simulink model "robot"  (R2017b)
settings: Solver=VariableStepAuto  StartTime=0.0  StopTime=10.0  RelTol=1e-3
libraries: vexarmcortexlib x16
settings Model: Creator=Chase B  LastModifiedBy=Chase B

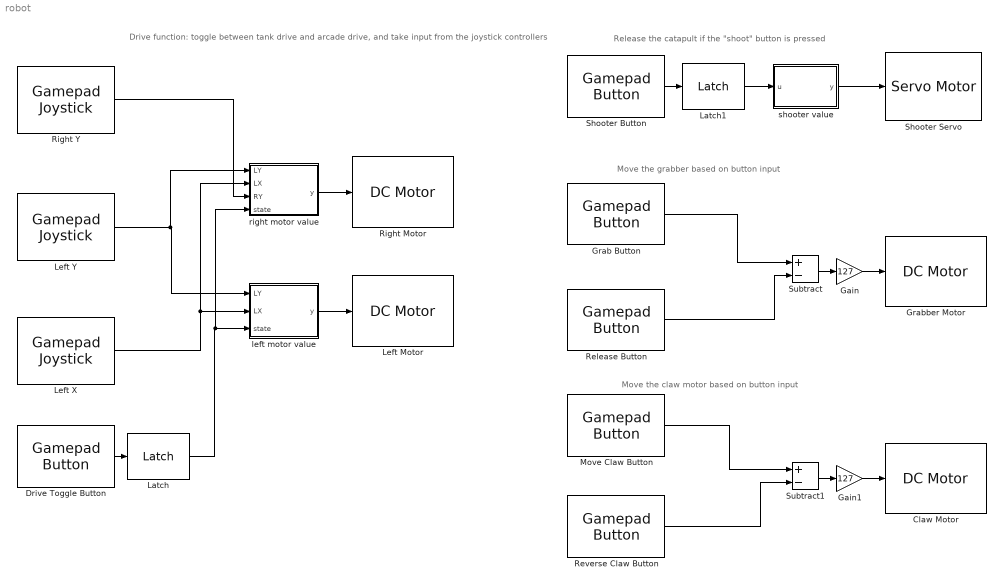
== system robot ==
  note: Move the claw motor based on button input
  note: Move the grabber based on button input
  note: Release the catapult if the "shoot" button is pressed
  note: Drive function: toggle between tank drive and arcade drive, and take input from the joystick controllers
  Claw Motor : vexarmcortexlib/Actuators/DC Motor  motor=8  scaleFactor=1/13.5  SimulationOut=off
      settings: SourceProductName=Simulink Coder Support Package for ARM Cortex-based VEX Microcontroller  SourceProductBaseCode=EC_VEX_MICRO
  Drive Toggle Button : vexarmcortexlib/Gamepad/Gamepad Button  joystick=1  chan=5  button56=Up  button78=Down  SimulationIn=off  SampleTime=0.2
      settings: SourceProductName=Simulink Coder Support Package for ARM Cortex-based VEX Microcontroller  SourceProductBaseCode=EC_VEX_MICRO
  Gain : Gain  Gain=127
  Gain1 : Gain  Gain=127
  Grab Button : vexarmcortexlib/Gamepad/Gamepad Button  joystick=1  chan=6  button56=Up  button78=Up  SimulationIn=off  SampleTime=0.2
      settings: SourceProductName=Simulink Coder Support Package for ARM Cortex-based VEX Microcontroller  SourceProductBaseCode=EC_VEX_MICRO
  Grabber Motor : vexarmcortexlib/Actuators/DC Motor  motor=3  scaleFactor=1/13.5  SimulationOut=off
      settings: SourceProductName=Simulink Coder Support Package for ARM Cortex-based VEX Microcontroller  SourceProductBaseCode=EC_VEX_MICRO
  Latch : vexarmcortexlib/Utilities/Latch  output0=off
      settings: SourceProductName=Simulink Coder Support Package for ARM Cortex-based VEX Microcontroller  SourceProductBaseCode=EC_VEX_MICRO
  Latch1 : vexarmcortexlib/Utilities/Latch  output0=off
      settings: SourceProductName=Simulink Coder Support Package for ARM Cortex-based VEX Microcontroller  SourceProductBaseCode=EC_VEX_MICRO
  Left Motor : vexarmcortexlib/Actuators/DC Motor  motor=9  scaleFactor=1/13.5  SimulationOut=off
      settings: SourceProductName=Simulink Coder Support Package for ARM Cortex-based VEX Microcontroller  SourceProductBaseCode=EC_VEX_MICRO
  Left X : vexarmcortexlib/Gamepad/Gamepad Joystick  joystick=1  chan=4  SimulationIn=off  SampleTime=0.2
      settings: SourceProductName=Simulink Coder Support Package for ARM Cortex-based VEX Microcontroller  SourceProductBaseCode=EC_VEX_MICRO
  Left Y : vexarmcortexlib/Gamepad/Gamepad Joystick  joystick=1  chan=3  SimulationIn=off  SampleTime=0.2
      settings: SourceProductName=Simulink Coder Support Package for ARM Cortex-based VEX Microcontroller  SourceProductBaseCode=EC_VEX_MICRO
  Move Claw Button : vexarmcortexlib/Gamepad/Gamepad Button  joystick=1  chan=7  button56=Up  button78=Left  SimulationIn=off  SampleTime=0.2
      settings: SourceProductName=Simulink Coder Support Package for ARM Cortex-based VEX Microcontroller  SourceProductBaseCode=EC_VEX_MICRO
  Release Button : vexarmcortexlib/Gamepad/Gamepad Button  joystick=1  chan=6  button56=Down  button78=Up  SimulationIn=off  SampleTime=0.2
      settings: SourceProductName=Simulink Coder Support Package for ARM Cortex-based VEX Microcontroller  SourceProductBaseCode=EC_VEX_MICRO
  Reverse Claw Button : vexarmcortexlib/Gamepad/Gamepad Button  joystick=1  chan=7  button56=Up  button78=Right  SimulationIn=off  SampleTime=0.2
      settings: SourceProductName=Simulink Coder Support Package for ARM Cortex-based VEX Microcontroller  SourceProductBaseCode=EC_VEX_MICRO
  Right Motor : vexarmcortexlib/Actuators/DC Motor  motor=2  scaleFactor=1/13.5  SimulationOut=off
      settings: SourceProductName=Simulink Coder Support Package for ARM Cortex-based VEX Microcontroller  SourceProductBaseCode=EC_VEX_MICRO
  Right Y : vexarmcortexlib/Gamepad/Gamepad Joystick  joystick=1  chan=2  SimulationIn=off  SampleTime=0.2
      settings: SourceProductName=Simulink Coder Support Package for ARM Cortex-based VEX Microcontroller  SourceProductBaseCode=EC_VEX_MICRO
  Shooter Button : vexarmcortexlib/Gamepad/Gamepad Button  joystick=1  chan=8  button56=Up  button78=Up  SimulationIn=off  SampleTime=0.2
      settings: SourceProductName=Simulink Coder Support Package for ARM Cortex-based VEX Microcontroller  SourceProductBaseCode=EC_VEX_MICRO
  Shooter Servo : vexarmcortexlib/Actuators/Servo Motor  motor=4  scaleFactor=60/127  SimulationOut=off
      settings: SourceProductName=Simulink Coder Support Package for ARM Cortex-based VEX Microcontroller  SourceProductBaseCode=EC_VEX_MICRO
  Subtract : Sum  Inputs=+-
  Subtract1 : Sum  Inputs=+-
  left motor value : MATLAB Function  TreatAsAtomicUnit=on
  right motor value : MATLAB Function  TreatAsAtomicUnit=on
  shooter value : MATLAB Function  TreatAsAtomicUnit=on
  wires:
  Left Y/1 -> right motor value/1(LY), left motor value/1(LY)
  Left X/1 -> right motor value/2(LX), left motor value/2(LX)
  Drive Toggle Button/1 -> Latch/1
  Latch/1 -> right motor value/4(state), left motor value/3(state)
  left motor value/1(y) -> Left Motor/1
  Right Y/1 -> right motor value/3(RY)
  right motor value/1(y) -> Right Motor/1
  Shooter Button/1 -> Latch1/1
  Latch1/1 -> shooter value/1(u)
  shooter value/1(y) -> Shooter Servo/1
  Grab Button/1 -> Subtract/1
  Release Button/1 -> Subtract/2
  Subtract/1 -> Gain/1
  Gain/1 -> Grabber Motor/1
  Move Claw Button/1 -> Subtract1/1
  Reverse Claw Button/1 -> Subtract1/2
  Subtract1/1 -> Gain1/1
  Gain1/1 -> Claw Motor/1

== matlab function robot/right motor value ==
  data: LY input; y output; LX input; RY input; state input
function y = fcn(LY, LX, RY, state)
% if the state is zero (false), drive in tank drive, otherwise (1, true) in arcade
y = state * (LY - LX) / 2 + (~state) * (RY);

== matlab function robot/left motor value ==
  data: LY input; y output; LX input; state input
function y = fcn(LY, LX, state)
% if the state is zero (false), drive in tank drive, otherwise (1, true) in arcade
y = state * (LY + LX) / 2 + (~state) * (LY);

== matlab function robot/shooter value ==
  data: u input; y output
function y = fcn(u)
% if the state is zero, move the motor to position -128, otherwise 127
y = u*255 - 128;
